simulink model "Qpsk"  (R2018b)
settings: Solver=VariableStepAuto  StartTime=0.0  StopTime=5  MaxStep=0.001  RelTol=1e-3
libraries: simulink x2
settings Model: Creator=sin  LastModifiedBy=sin

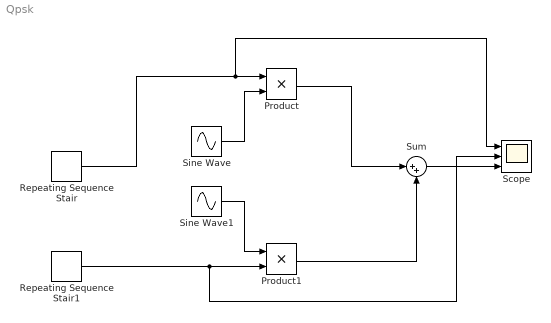
== system Qpsk ==
  Product : Product
  Product1 : Product
  Repeating Sequence Stair : simulink/Sources/Repeating Sequence Stair  OutValues=[-1 1 -1 1 -1].'  tsamp=1  OutMin=[]  OutMax=[]  OutDataTypeStr=double  OutputDataTypeScalingMode=double  OutDataType=fixdt(0,8)  ConRadixGroup=Best Precision: Vector-wise  OutScaling=2^-12
  Repeating Sequence Stair1 : simulink/Sources/Repeating Sequence Stair  OutValues=[-1 1 1 -1 1].'  tsamp=1  OutMin=[]  OutMax=[]  OutDataTypeStr=double  OutputDataTypeScalingMode=double  OutDataType=fixdt(0,8)  ConRadixGroup=Best Precision: Vector-wise  OutScaling=2^-12
  Scope : Scope  NumInputPorts=3
  Sine Wave : Sin  Amplitude=1/1.414  Frequency=2*2*pi  Phase=pi/2  SampleTime=0
  Sine Wave1 : Sin  Amplitude=1/1.414  Frequency=2*2*pi  SampleTime=0
  Sum : Sum  Inputs=|++
  wires:
  Repeating Sequence Stair/1 -> Scope/1, Product/1
  Repeating Sequence Stair1/1 -> Scope/2, Product1/2
  Sine Wave1/1 -> Product1/1
  Sine Wave/1 -> Product/2
  Product/1 -> Sum/1
  Product1/1 -> Sum/2
  Sum/1 -> Scope/3
